simulink model "wuty_PM"  (R2019a)
settings: Solver=FixedStepAuto  StartTime=0.0  StopTime=6000  RelTol=1e-3  EnableMultiTasking=on
libraries: arduinolib x7
settings Model: SnapshotBufferSize=100  SnapshotInterval=1  ExtModeTrigDuration=2  Creator=dell  LastModifiedBy=DELL-PC
settings SolverCC: PositivePriorityOrder=on  AutoInsertRateTranBlk=on
settings DataIOCC: LimitDataPoints=on  ReturnWorkspaceOutputs=off
settings OptimizationCC: EnhancedBackFolding=on  PassReuseOutputArgsAs=Individual arguments  ZeroExternalMemoryAtStartup=off  ZeroInternalMemoryAtStartup=off  MaxStackSize=64  OptimizeBlockOrder=speed  DifferentSizesBufferReuse=on  OptimizationCustomize=off
settings DebuggingCC: ParameterTunabilityLossMsg=error  AllowSymbolicDim=off  SFUnexpectedBacktrackingDiag=warning  SFNoUnconditionalDefaultTransitionDiag=warning  SFExecutionAtInitializationDiag=none  ArithmeticOperatorsInVariantConditions=warning
settings HardwareCC: ProdBitPerInt=16  ProdBitPerPointer=16  ProdBitPerSizeT=16  ProdBitPerPtrDiffT=16  ProdLargestAtomicFloat=None  ProdWordSize=8  ProdHWDeviceType=Atmel->AVR  UseEmbeddedCoderFeatures=off
settings SFSimCC: SimUseLocalCustomCode=off  MATLABDynamicMemAlloc=off
settings RTWCC: SystemTargetFile=ert.tlc  HardwareBoard=Arduino Uno  TLCOptions=-aInlineSetEventsForThisBaseRateFcn=TLC_FALSE -aSuppressMultiTaskScheduler=TLC_FALSE -aRateBasedStepFcn=1  TemplateMakefile=ert_default_tmf  GenerateReport=on  RTWUseLocalCustomCode=off  Toolchain=Arduino AVR  BuildConfiguration=Faster Runs  IncludeHyperlinkInReport=on  LaunchReport=on  GenerateTraceInfo=on  GenerateTraceReport=on  GenerateTraceReportSl=on  GenerateTraceReportSf=on  GenerateTraceReportEml=on
settings CodeAppCC: ForceParamTrailComments=on  IgnoreCustomStorageClasses=off  OperatorAnnotations=on  SimulinkDataObjDesc=on  SFDataObjDesc=on  InsertBlockDesc=on
settings ERTTargetCC: SupportContinuousTime=on  SupportNonInlinedSFcns=on  SupportVariableSizeSignals=on  ExtModeStaticAllocSize=250
settings ConfigComp: CovMetricSettings=dw  CovHtmlReporting=on  CovSaveCumulativeToWorkspaceVar=on  CovSaveSingleToWorkspaceVar=on  CovShowResultsExplorer=off  CovExternalEMLEnable=off

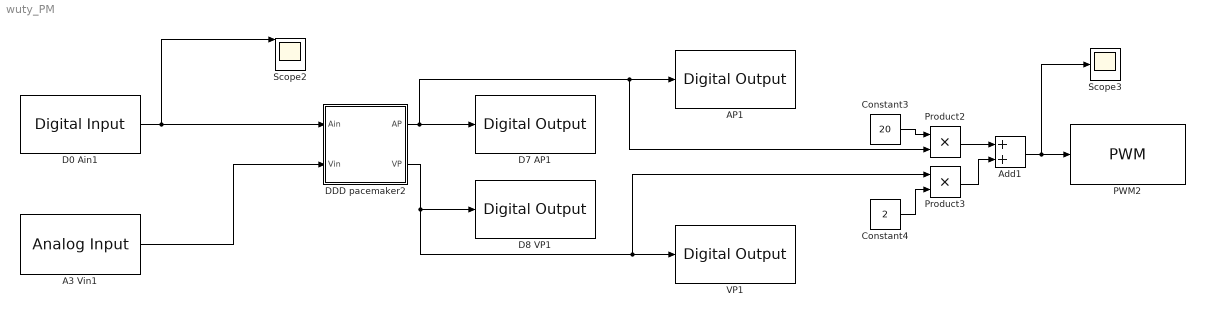
== system wuty_PM ==
  A3 Vin1 : arduinolib/Analog Input  pinNumber=3  ReadResultsOnly=off  ConversionTriggerSource=Software  ExternalTriggerType=uint32(0)  OutputDataType=uint16  EnableConversionCompleteNotify=off  EnableOuputStatus=off  SampleTime=inf  blockPlatform=arduino
  AP1 : arduinolib/Digital Output  pinNumber=13  blockPlatform=arduino
  Add1 : Sum
  Constant3 : Constant  Value=20
  Constant4 : Constant  Value=2
  D0 Ain1 : arduinolib/Digital Input  pinNumber=0  SampleTime=inf  blockPlatform=arduino
      settings: SourceProductName=Simulink Support Package for Arduino Hardware
  D7 AP1 : arduinolib/Digital Output  pinNumber=7  blockPlatform=arduino
  D8 VP1 : arduinolib/Digital Output  pinNumber=8  blockPlatform=arduino
  DDD pacemaker2 : Subsystem
  PWM2 : arduinolib/PWM  pinNumber=5  EnableInputFrequency=off  InitialFrequency=2000  InitialDutyCycle=0  NotificationType=None  blockPlatform=arduino
  Product2 : Product
  Product3 : Product
  Scope2 : Scope  NumInputPorts=4
  Scope3 : Scope
  VP1 : arduinolib/Digital Output  pinNumber=12  blockPlatform=arduino
  wires:
  Constant4/1 -> Product3/2
  Add1/1 -> Scope3/1, PWM2/1
  Constant3/1 -> Product2/1
  Product3/1 -> Add1/2
  D0 Ain1/1 -> Scope2/1, DDD pacemaker2/1(Ain)
  Product2/1 -> Add1/1
  DDD pacemaker2/1(AP) -> Product2/2, AP1/1, D7 AP1/1
  DDD pacemaker2/2(VP) -> D8 VP1/1, Product3/1, VP1/1
  A3 Vin1/1 -> DDD pacemaker2/2(Vin)

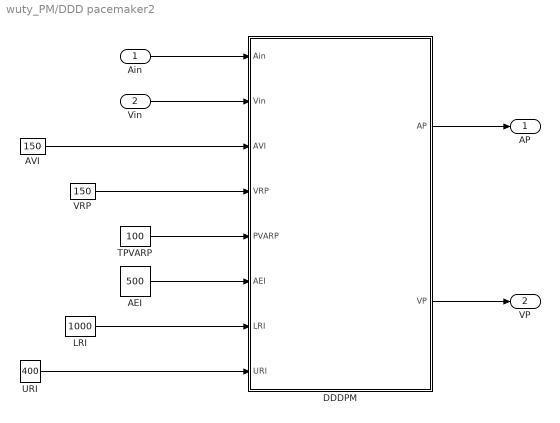
== system wuty_PM/DDD pacemaker2 ==
  Ain : Inport
  Vin : Inport  Port=2
  AEI : Constant  Value=500
  AVI : Constant  Value=150  OutDataTypeStr=uint16
  DDDPM : Stateflow chart  TreatAsAtomicUnit=on
  LRI : Constant  Value=1000  OutDataTypeStr=uint16
  TPVARP : Constant  Value=100  OutDataTypeStr=uint16
  URI : Constant  Value=400  OutDataTypeStr=uint16
  VRP : Constant  Value=150  OutDataTypeStr=uint16
  AP : Outport
  VP : Outport  Port=2
  wires:
  DDDPM/2(VP) -> VP/1
  DDDPM/1(AP) -> AP/1
  Vin/1 -> DDDPM/2(Vin)
  Ain/1 -> DDDPM/1(Ain)
  AVI/1 -> DDDPM/3(AVI)
  VRP/1 -> DDDPM/4(VRP)
  TPVARP/1 -> DDDPM/5(PVARP)
  URI/1 -> DDDPM/8(URI)
  LRI/1 -> DDDPM/7(LRI)
  AEI/1 -> DDDPM/6(AEI)

== stateflow chart wuty_PM/DDD pacemaker2/DDDPM ==
  settings: updateMethod=DISCRETE  sampleTime=1
  state DDDPM
    state AVI [parallel]
      settings: executionOrder=3
      state ActiveAVI
      state CAVI
      state IdleAVI
      (default) -> IdleAVI : {VP=false,VP1=false;}
      ActiveAVI -> ActiveAVI [order 3] : [tmpAVI>0]/{tmpAVI=tmpAVI-1;}
      IdleAVI -> ActiveAVI : [AS==true || AP1==true]/
          | {tmpAVI=AVI;}
      ActiveAVI -> CAVI [order 1] : [tmpAVI<=0&&enterURI==true]/
          | {VP=true, VP1=true;}
      ActiveAVI -> IdleAVI [order 2] : [VS==true || VP1==true]
      CAVI -> IdleAVI : {VP=false,VP1=false;}
    state URI [parallel]
      settings: executionOrder=1
      state IdleURI
      state ActiveURI
      (default) -> IdleURI : {enterURI=true;}
      IdleURI -> ActiveURI : [VP1==true || VS==true]/
          | {tmpURI=URI, enterURI=false;}
      ActiveURI -> IdleURI [order 3] : [tmpURI<=0]/{enterURI=true;}
      ActiveURI -> ActiveURI [order 2] : [tmpURI>0]/{tmpURI = tmpURI - 1;}
      ActiveURI -> ActiveURI [order 1] : [VS==true || VP1==true]/
          | {tmpURI=URI, enterURI=false;}
    state PVARP [parallel]
      settings: executionOrder=5
      state AinPVARP
      state IdlePVARP
      state ActivePVARP
      state PVARPAR
      IdlePVARP -> AinPVARP [order 1] : [Ain==true]/{AS=true}
      AinPVARP -> IdlePVARP : {AS=false;}
      (default) -> IdlePVARP : {AS=false;}
      IdlePVARP -> ActivePVARP [order 2] : [VS==true || VP1==true]/{tmpPVARP=PVARP;}
      ActivePVARP -> IdlePVARP [order 3] : [tmpPVARP<=0]
      ActivePVARP -> ActivePVARP [order 2] : [tmpPVARP>0]/
          | {tmpPVARP = tmpPVARP - 1;}
      PVARPAR -> ActivePVARP : {AR=false,tmpPVARP = tmpPVARP - 1;}
      ActivePVARP -> PVARPAR [order 1] : [Ain==true]/{AR=true;}
    state LRI [parallel]
      settings: executionOrder=2
      state IdleLRI
      state LRIVP
      state ActiveLRI
      IdleLRI -> IdleLRI [order 1] : [VS==true||VP1==true]/
          | {tmpLRI=LRI;}
      (default) -> IdleLRI : {tmpLRI = LRI,APLRI=2,AP=false,AP1=false;}
      IdleLRI -> IdleLRI [order 3] : [tmpLRI>AVI]/
          | {tmpLRI = tmpLRI-1;}
      LRIVP -> IdleLRI : /{VP=false, VP1=false, tmpLRI=LRI;}
      IdleLRI -> ActiveLRI [order 4] : [tmpLRI<=AVI]/
          | {AP=true,APLRI=1,AP1=true,tmpLRI=tmpLRI-1;}
      IdleLRI -> ActiveLRI [order 2] : [AS==true]/{tmpLRI=tmpLRI-1;}
      ActiveLRI -> IdleLRI [order 2] : [VS==true || VP1==true]/{tmpLRI=LRI;}
      ActiveLRI -> LRIVP [order 4] : [tmpLRI<=0]/
          | {VP=true,VP1=true;}
      ActiveLRI -> ActiveLRI [order 3] : [tmpLRI>0]
          | /{tmpLRI=tmpLRI-1;}
      ActiveLRI -> ActiveLRI [order 1] : [APLRI==1]/
          | {APLRI=APLRI+1,AP=false,AP1=false,
          | tmpLRI=tmpLRI-1;}
    state VRP [parallel]
      settings: executionOrder=4
      state VRPVS
      state IdleVRP
      state ActiveVRP
      IdleVRP -> VRPVS [order 1] : [Vin==true]/{VS=true}
      VRPVS -> ActiveVRP : {tmpVRP=VRP,VS=false;}
      (default) -> IdleVRP : {VS=false}
      IdleVRP -> ActiveVRP [order 2] : [VP1==true]/{tmpVRP=VRP;}
      ActiveVRP -> ActiveVRP [order 1] : [tmpVRP>0]/{tmpVRP= tmpVRP - 1;}
      ActiveVRP -> IdleVRP [order 2] : [tmpVRP<=0]
  (default) -> DDDPM : {VS=false, VP1=false, VP=false, AS=false,AR=false,AP1=false,  APLRI=2,  AP=false,  enterURI=true, tmpVRP=VRP, tmpPVARP = PVARP, tmpAVI= AVI, tmpLRI = LRI, tmpURI = URI;}
  data: Ain input; VS local; Vin input; AP output; VP output; tmpVRP local; AS local; tmpPVARP local; tmpAVI local; enterURI local; tmpLRI local; tmpURI local; APLRI local; VP1 local; AP1 local; AR local; AVI input uint16; VRP input uint16 =150; PVARP input uint16; AEI input; LRI input uint16; URI input uint16; APLRI1 local
